simulink model "BatterySimulation"  (R2018b)
settings: Solver=VariableStepAuto  StartTime=0.0  StopTime=10.0  RelTol=1e-3
libraries: canoelib x7
settings Model: Creator=jackb  LastModifiedBy=jackb

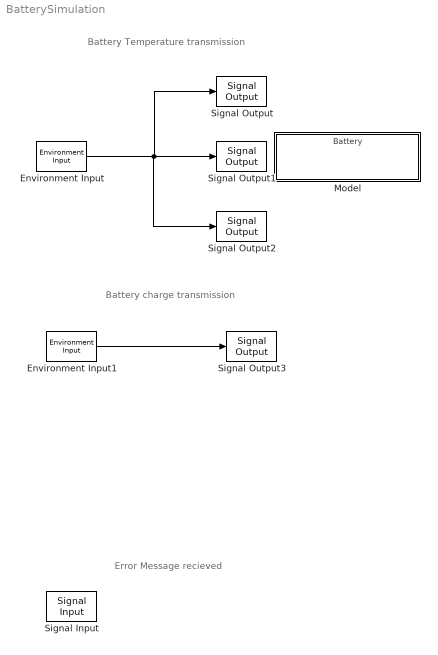
== system BatterySimulation ==
  note: Error Message recieved
  note: Battery Temperature transmission
  note: Battery charge transmission
  Environment Input : canoelib/CANoe I//O/Environment Input  envName=Battery_temp  editSampleTime=0  dataType=Default  dataTypeDB=int32
      settings: AttributesFormatString=%<envName>  SourceProductName=Vector CANoe
  Environment Input1 : canoelib/CANoe I//O/Environment Input  envName=Battery_temp  editSampleTime=0  dataType=Default  dataTypeDB=int32
      settings: AttributesFormatString=%<envName>  SourceProductName=Vector CANoe
  Model : ModelReference  ModelNameDialog=Battery.slx  SimulationMode=Normal  ModelReferenceVersion=1.2
  Signal Input : canoelib/CANoe I//O/Signal Input  dbName=0  nodeName=0  msgName=0  sigName=0  editSampleTime=0  rawValue=Default  dataType=Default  dataTypeDB=unknown  hasEncoding=off
      settings: AttributesFormatString=%<sigName>  SourceProductName=Vector CANoe
  Signal Output : canoelib/CANoe I//O/Signal Output  dbName=V2CANdb  nodeName=Battery  msgName=Bat_ActualValues  sigName=bat_temp1  rawValue=Default  dataType=Default  dataTypeDB=int8  hasEncoding=off
      settings: AttributesFormatString=%<sigName>  SourceProductName=Vector CANoe
  Signal Output1 : canoelib/CANoe I//O/Signal Output  dbName=V2CANdb  nodeName=Battery  msgName=Bat_ActualValues  sigName=bat_temp2  rawValue=Default  dataType=Default  dataTypeDB=int8  hasEncoding=off
      settings: AttributesFormatString=%<sigName>  SourceProductName=Vector CANoe
  Signal Output2 : canoelib/CANoe I//O/Signal Output  dbName=V2CANdb  nodeName=Battery  msgName=Bat_ActualValues  sigName=bat_temp3  rawValue=Default  dataType=Default  dataTypeDB=int8  hasEncoding=off
      settings: AttributesFormatString=%<sigName>  SourceProductName=Vector CANoe
  Signal Output3 : canoelib/CANoe I//O/Signal Output  dbName=V2CANdb  nodeName=Battery  msgName=Bat_ActualValues  sigName=bat_temp2  rawValue=Default  dataType=Default  dataTypeDB=int8  hasEncoding=off
      settings: AttributesFormatString=%<sigName>  SourceProductName=Vector CANoe
  wires:
  Environment Input/1 -> Signal Output2/1, Signal Output/1, Signal Output1/1
  Environment Input1/1 -> Signal Output3/1
